simulink model "consigna_5_2"  (R2024b)
settings: Solver=ode45  StartTime=0.0  StopTime=600  FixedStep=1/39789  MaxStep=1e-1  RelTol=1e-5
InitFcn:
  | parametros
values from neighbouring files (symbols this model uses):
  A_corrientes = [0 1; -omega_n_corrientes^2 -2*omega_n_corrientes]    [parametros.m]
  A_inversor = [0 1; -omega_n_inversor^2 -2*omega_n_inversor]    [parametros.m]
  A_posicion = [0 1; -omega_n_posicion^2 -2*omega_n_posicion]    [parametros.m]
  A_temp = -1/20    (= -0.05)    [parametros.m]
  alpha_cu = 3.9 *10^-3    (= 0.0039)    [parametros.m]
  B_corrientes = [0; omega_n_corrientes^2]    [parametros.m]
  B_inversor = [0; omega_n_inversor^2]    [parametros.m]
  b_l = 0.1    [parametros.m]
  b_m = 1.5 * 10^-5    (= 1.5e-05)    [parametros.m]
  B_posicion = [0; omega_n_posicion^2]    [parametros.m]
  B_temp = 1/20    (= 0.05)    [parametros.m]
  ba = J_eq*n*omega_pos    (= 0.0395694444444)    [parametros.m]
  C_corrientes = [1 0]    [parametros.m]
  C_inversor = [1 0]    [parametros.m]
  C_posicion = [1 0]    [parametros.m]
  C_temp = 1    [parametros.m]
  C_ts = 0.818    [parametros.m]
  J_l = (m*l_cm^2 + J_cm) + (m_l * l_l^2)    (= 0.0833)    [parametros.m]
  J_m = 1.4 * 10^-5    (= 1.4e-05)    [parametros.m]
  K_e_int = 3200 ^3    (= 32768000000)    [parametros.m]
  K_e_omega = 3*3200^2    (= 30720000)    [parametros.m]
  K_e_theta = 9600    [parametros.m]
  k_l = m * g * l_cm + m_l * g * l_l    (= 2.4516625)    [parametros.m]
  Ksa = J_eq*n*(omega_pos^2)    (= 31.6555555556)    [parametros.m]
  Ksia = J_eq*(omega_pos^3)    (= 10129.7777778)    [parametros.m]
  L_d = 6.6 * 10^-3    (= 0.0066)    [parametros.m]
  L_ls = 0.8 * 10^-3    (= 0.0008)    [parametros.m]
  L_q = 5.8 * 10^-3    (= 0.0058)    [parametros.m]
  lambda_m = 0.016    [parametros.m]
  P_p = 3    [parametros.m]
  r = 120    [parametros.m]
  R_s_40 = 1.02    [parametros.m]
  R_ts_amb = 146.7    [parametros.m]
  T_sample = 1/f_sample    (= 4.53514739229e-05)    [parametros.m]
  Temp_s_ref = 20    [parametros.m]
  tm = X(1)    [parametros.m]
  tr = X(2)    [parametros.m]
  w1 = 2*pi*r/5    (= 150.796447372)    [parametros.m]
  x0_corrientes = [0;0]    [parametros.m]
  x0_inversor = [0;0]    [parametros.m]
  x0_posicion = [0; 0]    [parametros.m]
  x0_temp = 25    [parametros.m]
libraries: simulink x23, dspsigops x6
(part 2 of 5)

== system consigna_5_2/5.2.5.c ==
  note: CONTROLADOR
  T_per : Inport
  Tº_amb : Inport  Port=2
  q1* : Inport  Port=3
  Calculo rs : Subsystem
  Constant5 : Constant  Value=0
  Controlador PID : Subsystem
  Demux : Demux  Outputs=3
  Desacoplamiento de torque de gravedad : Subsystem
  Desacoplamientos físicos : Subsystem
  Gain5 : Gain  Gain=P_p
  Inversión de tensión : Subsystem
  Modulador de corriente : Subsystem
  Modulador de torque : Subsystem
  Mux : Mux  Inputs=3
  Mux1 : Mux  Inputs=2
  Observador de estado reducido : Subsystem
  Sensores : Subsystem
  Setpoint : Subsystem
  Subsistema físico no lineal : Subsystem
      settings: PortSchema="{\"entries\":[{\"content\":{\"sides\":[{\"content\":{\"connectorIds\":[\"In1\",\"In2\",\"In3\",\"In4\",\"In5\"]},\"type\":\"ConnectorPlacement.EquallySpacedRectSide\",\"uuid\":\"67117692-d9ee-40bf-88b2-d8f6a60dc3b5\"},{\"content\":{\"connectorIds\":[\"Out1\",\"Out2\",\"Out3\"],\"side\":\"RIGHT\"},\"type\":\"ConnectorPlacement.EquallySpacedRectSide\",\"uuid\":\"ca2dbe86-e86f-47c7-8eac-1e82e6a5dbc0\"},{\"content\":{\"connectorIds\":[\"Out4\",\"Out5\",\"Out6\"],\"side\":\"TOP\"},\"type\":\"ConnectorPlacement.EquallySpacedRectSide\",\"uuid\":\"fbd4a5c3-5162-48dd-8002-932f8e6631f6\"}]},\"type\":\"ConnectorPlacement.EquallySpacedConnector\",\"uuid\":\"e55c07f0-88b9-4508-920f-2bf50421126b\"}],\"packageUris\":[\"http://schema.mathworks.com/mf0/Connector/R2020b\"],\"version\":\"1.0\"}"
  TD_PARK : MATLAB Function  TreatAsAtomicUnit=on
  TI_PARK1 : MATLAB Function  TreatAsAtomicUnit=on
  T_l : Outport
  T_m : Outport  Port=2
  "theta_m " : Outport  Port=3
  T_s : Outport  Port=4
  fas : Outport  Port=5
  fbs : Outport  Port=6
  fcs : Outport  Port=7
  v_abcs : Outport  Port=8
  omega_m : Outport  Port=9
  omega_theta_obs : Outport  Port=10
  wires:
  Inversión de tensión/1(v_as) -> Subsistema físico no lineal/2(v_as), Mux/1
  TD_PARK/3(f0s) -> Modulador de corriente/6(i_0s), Desacoplamientos físicos/6(i_0s)  "i_0s"
  TI_PARK1/1(fas) -> Inversión de tensión/1(v_as*)
  Inversión de tensión/2(v_bs) -> Mux/2, Subsistema físico no lineal/3(v_bs)
  TD_PARK/1(fqs) -> Modulador de corriente/4(i_qs), Desacoplamientos físicos/4(i_qs)  "i_qs^r"
  Gain5/1 -> TD_PARK/4(theta_r), TI_PARK1/4(theta_r)
  TI_PARK1/2(fbs) -> Inversión de tensión/2(v_bs*)
  TD_PARK/2(fds) -> Modulador de torque/2(ids), Modulador de corriente/5(i_ds), Desacoplamientos físicos/5(i_ds)  "i_ds^r"
  Desacoplamientos físicos/3(v_0s*') -> TI_PARK1/3(f0s)
  Inversión de tensión/3(v_cs) -> Mux/3, Subsistema físico no lineal/4(v_cs)
  Subsistema físico no lineal/1(theta_m) -> Sensores/1(theta_m)
  Subsistema físico no lineal/2(T_s) -> Sensores/2(T_s)
  Sensores/5(i_cs_medida) -> fcs/1, TD_PARK/3(fcs)
  Demux/1 -> Sensores/3(i_as)
  Modulador de torque/1(iq*) -> Modulador de corriente/1(I_qs*)
  Sensores/4(i_bs_medida) -> fbs/1, TD_PARK/2(fbs)
  Subsistema físico no lineal/5(T_m) -> T_m/1
  Modulador de corriente/1(v_qs*) -> Desacoplamientos físicos/1(v_qs*)
  Constant5/1 -> Modulador de corriente/3(I_0s*), Modulador de corriente/2(I_ds*)
  T_per/1 -> Subsistema físico no lineal/1(T_per)
  Demux/2 -> Sensores/4(i_bs)
  Modulador de corriente/3(v_0s*) -> Desacoplamientos físicos/3(v_0s*)
  Demux/3 -> Sensores/5(i_cs)
  Sensores/1(theta_m_medida) -> "theta_m "/1, Observador de estado reducido/2(theta_m), Gain5/1
  Desacoplamientos físicos/1(v_qs*') -> TI_PARK1/1(fqs)
  Sensores/3(i_as_medida) -> TD_PARK/1(fas), fas/1
  TI_PARK1/3(fcs) -> Inversión de tensión/3(v_cs*)
  Desacoplamientos físicos/2(v_ds*') -> TI_PARK1/2(fds)
  Modulador de corriente/2(v_ds*) -> Desacoplamientos físicos/2(v_ds*)
  Setpoint/2(omega_m*) -> Controlador PID/1(omega_m*)
  q1*/1 -> Setpoint/1(q1*)
  Controlador PID/1(Tm*) -> Observador de estado reducido/1(T_m*), Desacoplamiento de torque de gravedad/1(Tm*)
  Tº_amb/1 -> Subsistema físico no lineal/5(Tº_amb)
  Sensores/2(T_s_medida) -> Calculo rs/1(Ts), T_s/1
  Calculo rs/1(r_s) -> Desacoplamientos físicos/8(r_s)
  Desacoplamiento de torque de gravedad/1(Tm*') -> Modulador de torque/1(Tm*)
  Mux/1 -> v_abcs/1
  Subsistema físico no lineal/4(omega_m) -> omega_m/1  "omega_m"
  Mux1/1 -> omega_theta_obs/1
  Observador de estado reducido/2(theta_m_obs) -> Mux1/2, Desacoplamiento de torque de gravedad/2(theta_m)
  Observador de estado reducido/1(omega_m_obs) -> Mux1/1, Modulador de torque/3(omega_m), Controlador PID/2(omega_m), Desacoplamientos físicos/7(omega_m)
  Subsistema físico no lineal/6(T_l) -> T_l/1
  Subsistema físico no lineal/3(i_abcs) -> Demux/1

== system consigna_5_2/5.2.5.d ==
  note: CONTROLADOR
  T_per : Inport
  Tº_amb : Inport  Port=2
  q1* : Inport  Port=3
  Calculo rs : Subsystem
  Constant5 : Constant  Value=0
  Controlador PID : Subsystem
  Demux : Demux  Outputs=3
  Desacoplamiento de torque de gravedad : Subsystem
  Desacoplamientos físicos : Subsystem
  Gain5 : Gain  Gain=P_p
  Inversión de tensión : Subsystem
  Modulador de corriente : Subsystem
  Modulador de torque : Subsystem
  Mux : Mux  Inputs=3
  Mux1 : Mux  Inputs=2
  Observador de estado reducido : Subsystem
  Sensores : Subsystem
  Setpoint : Subsystem
  Subsistema físico no lineal : Subsystem
      settings: PortSchema="{\"entries\":[{\"content\":{\"sides\":[{\"content\":{\"connectorIds\":[\"In1\",\"In2\",\"In3\",\"In4\",\"In5\"]},\"type\":\"ConnectorPlacement.EquallySpacedRectSide\",\"uuid\":\"67117692-d9ee-40bf-88b2-d8f6a60dc3b5\"},{\"content\":{\"connectorIds\":[\"Out1\",\"Out2\",\"Out3\"],\"side\":\"RIGHT\"},\"type\":\"ConnectorPlacement.EquallySpacedRectSide\",\"uuid\":\"ca2dbe86-e86f-47c7-8eac-1e82e6a5dbc0\"},{\"content\":{\"connectorIds\":[\"Out4\",\"Out5\",\"Out6\"],\"side\":\"TOP\"},\"type\":\"ConnectorPlacement.EquallySpacedRectSide\",\"uuid\":\"fbd4a5c3-5162-48dd-8002-932f8e6631f6\"}]},\"type\":\"ConnectorPlacement.EquallySpacedConnector\",\"uuid\":\"e55c07f0-88b9-4508-920f-2bf50421126b\"}],\"packageUris\":[\"http://schema.mathworks.com/mf0/Connector/R2020b\"],\"version\":\"1.0\"}"
  TD_PARK : MATLAB Function  TreatAsAtomicUnit=on
  TI_PARK1 : MATLAB Function  TreatAsAtomicUnit=on
  T_l : Outport
  T_m : Outport  Port=2
  "theta_m " : Outport  Port=3
  T_s : Outport  Port=4
  fas : Outport  Port=5
  fbs : Outport  Port=6
  fcs : Outport  Port=7
  v_abcs : Outport  Port=8
  omega_theta_obs : Outport  Port=9
  omega_m : Outport  Port=10
  wires:
  Inversión de tensión/1(v_as) -> Subsistema físico no lineal/2(v_as), Mux/1
  TD_PARK/3(f0s) -> Modulador de corriente/6(i_0s), Desacoplamientos físicos/6(i_0s)  "i_0s"
  TI_PARK1/1(fas) -> Inversión de tensión/1(v_as*)
  Inversión de tensión/2(v_bs) -> Subsistema físico no lineal/3(v_bs), Mux/2
  TD_PARK/1(fqs) -> Modulador de corriente/4(i_qs), Desacoplamientos físicos/4(i_qs)  "i_qs^r"
  Gain5/1 -> TD_PARK/4(theta_r), TI_PARK1/4(theta_r)
  TI_PARK1/2(fbs) -> Inversión de tensión/2(v_bs*)
  TD_PARK/2(fds) -> Modulador de torque/2(ids), Modulador de corriente/5(i_ds), Desacoplamientos físicos/5(i_ds)  "i_ds^r"
  Desacoplamientos físicos/3(v_0s*') -> TI_PARK1/3(f0s)
  Inversión de tensión/3(v_cs) -> Subsistema físico no lineal/4(v_cs), Mux/3
  Subsistema físico no lineal/1(theta_m) -> Sensores/1(theta_m)
  Subsistema físico no lineal/2(T_s) -> Sensores/2(T_s)
  Sensores/5(i_cs_medida) -> fcs/1, TD_PARK/3(fcs)
  Demux/1 -> Sensores/3(i_as)
  Modulador de torque/1(iq*) -> Modulador de corriente/1(I_qs*)
  Sensores/4(i_bs_medida) -> fbs/1, TD_PARK/2(fbs)
  Modulador de corriente/1(v_qs*) -> Desacoplamientos físicos/1(v_qs*)
  Constant5/1 -> Modulador de corriente/3(I_0s*), Modulador de corriente/2(I_ds*)
  T_per/1 -> Subsistema físico no lineal/1(T_per)
  Demux/2 -> Sensores/4(i_bs)
  Modulador de corriente/3(v_0s*) -> Desacoplamientos físicos/3(v_0s*)
  Demux/3 -> Sensores/5(i_cs)
  Sensores/1(theta_m_medida) -> "theta_m "/1, Observador de estado reducido/2(theta_m), Gain5/1
  Desacoplamientos físicos/1(v_qs*') -> TI_PARK1/1(fqs)
  Sensores/3(i_as_medida) -> TD_PARK/1(fas), fas/1
  TI_PARK1/3(fcs) -> Inversión de tensión/3(v_cs*)
  Desacoplamientos físicos/2(v_ds*') -> TI_PARK1/2(fds)
  Modulador de corriente/2(v_ds*) -> Desacoplamientos físicos/2(v_ds*)
  Setpoint/2(omega_m*) -> Controlador PID/1(omega_m*)
  q1*/1 -> Setpoint/1(q1*)
  Controlador PID/1(Tm*) -> Observador de estado reducido/1(T_m*), Desacoplamiento de torque de gravedad/1(Tm*)
  Tº_amb/1 -> Subsistema físico no lineal/5(Tº_amb)
  Sensores/2(T_s_medida) -> Calculo rs/1(Ts), T_s/1
  Calculo rs/1(r_s) -> Desacoplamientos físicos/8(r_s)
  Desacoplamiento de torque de gravedad/1(Tm*') -> Modulador de torque/1(Tm*)
  Mux/1 -> v_abcs/1
  Mux1/1 -> omega_theta_obs/1
  Observador de estado reducido/2(theta_m_obs) -> Mux1/2, Desacoplamiento de torque de gravedad/2(theta_m)
  Observador de estado reducido/1(omega_m_obs) -> Mux1/1, Modulador de torque/3(omega_m), Controlador PID/2(omega_m), Desacoplamientos físicos/7(omega_m)
  Subsistema físico no lineal/5(T_m) -> T_m/1
  Subsistema físico no lineal/4(omega_m) -> omega_m/1  "omega_m"
  Subsistema físico no lineal/3(i_abcs) -> Demux/1
  Subsistema físico no lineal/6(T_l) -> T_l/1

== system consigna_5_2/5.2.5.e ==
  note: CONTROLADOR
  T_per : Inport
  Tº_amb : Inport  Port=2
  q1* : Inport  Port=3
  Calculo rs : Subsystem
  Constant5 : Constant  Value=0
  Controlador PID : Subsystem
  Demux : Demux  Outputs=3
  Desacoplamiento de torque de gravedad : Subsystem
  Desacoplamientos físicos : Subsystem
  Gain5 : Gain  Gain=P_p
  Inversión de tensión : Subsystem
  Modulador de corriente : Subsystem
  Modulador de torque : Subsystem
  Mux : Mux  Inputs=3
  Mux1 : Mux  Inputs=2
  Observador de estado reducido : Subsystem
  Sensores : Subsystem
  Setpoint : Subsystem
  Subsistema físico no lineal : Subsystem
      settings: PortSchema="{\"entries\":[{\"content\":{\"sides\":[{\"content\":{\"connectorIds\":[\"In1\",\"In2\",\"In3\",\"In4\",\"In5\"]},\"type\":\"ConnectorPlacement.EquallySpacedRectSide\",\"uuid\":\"67117692-d9ee-40bf-88b2-d8f6a60dc3b5\"},{\"content\":{\"connectorIds\":[\"Out1\",\"Out2\",\"Out3\"],\"side\":\"RIGHT\"},\"type\":\"ConnectorPlacement.EquallySpacedRectSide\",\"uuid\":\"ca2dbe86-e86f-47c7-8eac-1e82e6a5dbc0\"},{\"content\":{\"connectorIds\":[\"Out4\",\"Out5\",\"Out6\"],\"side\":\"TOP\"},\"type\":\"ConnectorPlacement.EquallySpacedRectSide\",\"uuid\":\"fbd4a5c3-5162-48dd-8002-932f8e6631f6\"}]},\"type\":\"ConnectorPlacement.EquallySpacedConnector\",\"uuid\":\"e55c07f0-88b9-4508-920f-2bf50421126b\"}],\"packageUris\":[\"http://schema.mathworks.com/mf0/Connector/R2020b\"],\"version\":\"1.0\"}"
  TD_PARK : MATLAB Function  TreatAsAtomicUnit=on
  TI_PARK1 : MATLAB Function  TreatAsAtomicUnit=on
  T_l : Outport
  T_m : Outport  Port=2
  "theta_m " : Outport  Port=3
  T_s : Outport  Port=4
  fas : Outport  Port=5
  fbs : Outport  Port=6
  fcs : Outport  Port=7
  v_abcs : Outport  Port=8
  omega_theta_obs : Outport  Port=9
  omega_m : Outport  Port=10
  wires:
  Inversión de tensión/1(v_as) -> Subsistema físico no lineal/2(v_as), Mux/1
  TD_PARK/3(f0s) -> Modulador de corriente/6(i_0s), Desacoplamientos físicos/6(i_0s)  "i_0s"
  TI_PARK1/1(fas) -> Inversión de tensión/1(v_as*)
  Inversión de tensión/2(v_bs) -> Subsistema físico no lineal/3(v_bs), Mux/2
  TD_PARK/1(fqs) -> Modulador de corriente/4(i_qs), Desacoplamientos físicos/4(i_qs)  "i_qs^r"
  Gain5/1 -> TD_PARK/4(theta_r), TI_PARK1/4(theta_r)
  TI_PARK1/2(fbs) -> Inversión de tensión/2(v_bs*)
  TD_PARK/2(fds) -> Modulador de torque/2(ids), Modulador de corriente/5(i_ds), Desacoplamientos físicos/5(i_ds)  "i_ds^r"
  Desacoplamientos físicos/3(v_0s*') -> TI_PARK1/3(f0s)
  Inversión de tensión/3(v_cs) -> Subsistema físico no lineal/4(v_cs), Mux/3
  Subsistema físico no lineal/1(theta_m) -> Sensores/1(theta_m)
  Subsistema físico no lineal/2(T_s) -> Sensores/2(T_s)
  Sensores/5(i_cs_medida) -> fcs/1, TD_PARK/3(fcs)
  Modulador de torque/1(iq*) -> Modulador de corriente/1(I_qs*)
  Sensores/4(i_bs_medida) -> fbs/1, TD_PARK/2(fbs)
  Modulador de corriente/1(v_qs*) -> Desacoplamientos físicos/1(v_qs*)
  Constant5/1 -> Modulador de corriente/3(I_0s*), Modulador de corriente/2(I_ds*)
  T_per/1 -> Subsistema físico no lineal/1(T_per)
  Demux/2 -> Sensores/4(i_bs)
  Modulador de corriente/3(v_0s*) -> Desacoplamientos físicos/3(v_0s*)
  Demux/3 -> Sensores/5(i_cs)
  Sensores/1(theta_m_medida) -> "theta_m "/1, Observador de estado reducido/2(theta_m), Gain5/1
  Desacoplamientos físicos/1(v_qs*') -> TI_PARK1/1(fqs)
  Sensores/3(i_as_medida) -> TD_PARK/1(fas), fas/1
  TI_PARK1/3(fcs) -> Inversión de tensión/3(v_cs*)
  Desacoplamientos físicos/2(v_ds*') -> TI_PARK1/2(fds)
  Modulador de corriente/2(v_ds*) -> Desacoplamientos físicos/2(v_ds*)
  Setpoint/2(omega_m*) -> Controlador PID/1(omega_m*)
  q1*/1 -> Setpoint/1(q1*)
  Controlador PID/1(Tm*) -> Observador de estado reducido/1(T_m*), Desacoplamiento de torque de gravedad/1(Tm*)
  Tº_amb/1 -> Subsistema físico no lineal/5(Tº_amb)
  Sensores/2(T_s_medida) -> Calculo rs/1(Ts), T_s/1
  Calculo rs/1(r_s) -> Desacoplamientos físicos/8(r_s)
  Desacoplamiento de torque de gravedad/1(Tm*') -> Modulador de torque/1(Tm*)
  Mux/1 -> v_abcs/1
  Mux1/1 -> omega_theta_obs/1
  Observador de estado reducido/2(theta_m_obs) -> Mux1/2, Desacoplamiento de torque de gravedad/2(theta_m)
  Observador de estado reducido/1(omega_m_obs) -> Mux1/1, Modulador de torque/3(omega_m), Controlador PID/2(omega_m), Desacoplamientos físicos/7(omega_m)
  Subsistema físico no lineal/5(T_m) -> T_m/1
  Subsistema físico no lineal/6(T_l) -> T_l/1
  Subsistema físico no lineal/4(omega_m) -> omega_m/1  "omega_m"
  Subsistema físico no lineal/3(i_abcs) -> Demux/1
  Demux/1 -> Sensores/3(i_as)

== system consigna_5_2/Subsystem ==
  T_per : Inport
  Tº_amb : Inport  Port=2
  q1* : Inport  Port=3
  5.2.6 : Subsystem
  omega_m : Outport
  Tm : Outport  Port=2
  theta_m : Outport  Port=3
  T_s : Outport  Port=4
  i_as : Outport  Port=5
  i_bs : Outport  Port=6
  i_cs : Outport  Port=7
  v_abcs : Outport  Port=8
  omega_theta_obs : Outport  Port=9
  omega_m1 : Outport  Port=10
  wires:
  q1*/1 -> 5.2.6/3(q1*)
  5.2.6/3("theta_m ") -> theta_m/1  "theta_m"
  T_per/1 -> 5.2.6/1(T_per)
  5.2.6/1(T_l) -> omega_m/1  "omega_m"
  5.2.6/4(T_s) -> T_s/1  "T_s"
  5.2.6/2(T_m) -> Tm/1  "Tm"
  5.2.6/5(fas) -> i_as/1  "i_as"
  5.2.6/10(omega_m) -> omega_m1/1  "omega_m"
  5.2.6/9(omega_theta_obs) -> omega_theta_obs/1
  5.2.6/7(fcs) -> i_cs/1  "i_cs"
  Tº_amb/1 -> 5.2.6/2(Tº_amb)
  5.2.6/6(fbs) -> i_bs/1  "i_bs"
  5.2.6/8(v_abcs) -> v_abcs/1

== system consigna_5_2/5.2.1 /Calculo rs ==
  Ts : Inport
  Tamb : Inport  Port=2
  Constant : Constant
  Gain : Gain  Gain=alpha_cu
  Gain1 : Gain  Gain=R_s_40
  Sum : Sum  Inputs=|++
  Sum1 : Sum  Inputs=|-+
  r_s : Outport
  wires:
  Constant/1 -> Sum/1
  Gain/1 -> Sum/2
  Ts/1 -> Sum1/2
  Tamb/1 -> Sum1/1
  Sum1/1 -> Gain/1
  Sum/1 -> Gain1/1
  Gain1/1 -> r_s/1

== system consigna_5_2/5.2.1 /Desacoplamientos físicos ==
  v_qs* : Inport
  v_ds* : Inport  Port=2
  v_0s* : Inport  Port=3
  i_qs : Inport  Port=4
  i_ds : Inport  Port=5
  i_0s : Inport  Port=6
  omega_m : Inport  Port=7
  r_s : Inport  Port=8
  Constant : Constant  Value=lambda_m
  Gain : Gain  Gain=P_p
  Gain1 : Gain  Gain=L_d
  Gain2 : Gain  Gain=L_q*P_p
  Product{,1..4} (5 alike) : Product
  Sum : Sum  Inputs=|++
  Sum1 : Sum  Inputs=|++
  Sum2 : Sum  Inputs=++|
  Sum3 : Sum  Inputs=+-|
  Sum4 : Sum  Inputs=|++
  Sum5 : Sum  Inputs=++|
  v_qs*' : Outport
  v_ds*' : Outport  Port=2
  v_0s*' : Outport  Port=3
  wires:
  Product/1 -> Sum/2
  r_s/1 -> Product4/1, Product/1, Product2/1
  i_qs/1 -> Product/2, Gain2/1
  v_qs*/1 -> Sum/1
  Sum/1 -> Sum1/1
  omega_m/1 -> Product3/2, Gain/1
  Product1/1 -> Sum1/2
  Gain/1 -> Product1/2
  i_ds/1 -> Gain1/1, Product2/2
  Gain1/1 -> Sum2/2
  Constant/1 -> Sum2/1
  Sum2/1 -> Product1/1
  Sum1/1 -> v_qs*'/1
  Product2/1 -> Sum3/1
  Gain2/1 -> Product3/1
  Product3/1 -> Sum3/2
  Sum3/1 -> Sum4/2
  v_ds*/1 -> Sum4/1
  Sum4/1 -> v_ds*'/1
  i_0s/1 -> Product4/2
  Product4/1 -> Sum5/1
  v_0s*/1 -> Sum5/2
  Sum5/1 -> v_0s*'/1

== system consigna_5_2/5.2.1 /Desacoplamientos físicos de torque ==
  Tm* : Inport
  theta_m : Inport  Port=2
  Gain : Gain  Gain=k_l
  Gain1 : Gain  Gain=1/r
  Gain2 : Gain  Gain=1/r
  Sin : Trigonometry
  Sum : Sum  Inputs=|++
  Tm*' : Outport
  wires:
  Tm*/1 -> Sum/1
  theta_m/1 -> Gain1/1
  Sin/1 -> Gain/1
  Sum/1 -> Tm*'/1
  Gain1/1 -> Sin/1
  Gain/1 -> Gain2/1
  Gain2/1 -> Sum/2

== system consigna_5_2/5.2.1 /Modulador de corriente ==
  I_qs* : Inport
  I_ds* : Inport  Port=2
  I_0s* : Inport  Port=3
  i_qs : Inport  Port=4
  i_ds : Inport  Port=5
  i_0s : Inport  Port=6
  Gain : Gain  Gain=5000*L_q
  Gain1 : Gain  Gain=5000*L_d
  Gain2 : Gain  Gain=5000*L_ls
  Sum : Sum  Inputs=+-
  Sum1 : Sum  Inputs=+-
  Sum2 : Sum  Inputs=+-
  v_qs* : Outport
  v_ds* : Outport  Port=2
  v_0s* : Outport  Port=3
  wires:
  Sum2/1 -> Gain2/1
  Sum1/1 -> Gain1/1
  Sum/1 -> Gain/1
  I_qs*/1 -> Sum/1
  i_qs/1 -> Sum/2
  I_ds*/1 -> Sum1/1
  i_ds/1 -> Sum1/2
  I_0s*/1 -> Sum2/1
  i_0s/1 -> Sum2/2
  Gain/1 -> v_qs*/1
  Gain2/1 -> v_0s*/1
  Gain1/1 -> v_ds*/1

== system consigna_5_2/5.2.1 /Modulador de tensión ==
  v_as* : Inport
  v_bs* : Inport  Port=2
  v_cs* : Inport  Port=3
  Gain : Gain
  Gain1 : Gain
  Gain2 : Gain
  v_as : Outport
  v_bs : Outport  Port=2
  v_cs : Outport  Port=3
  wires:
  v_as*/1 -> Gain/1
  Gain/1 -> v_as/1
  v_bs*/1 -> Gain1/1
  Gain1/1 -> v_bs/1
  v_cs*/1 -> Gain2/1
  Gain2/1 -> v_cs/1

== system consigna_5_2/5.2.1 /Modulador de torque ==
  Tm* : Inport
  ids : Inport  Port=2
  omega_m : Inport  Port=3
  Constant : Constant  Value=lambda_m
  Divide : Product  Inputs=/*
  Gain : Gain  Gain=b_m + b_l/r^2
  Gain1 : Gain  Gain=2/(3*P_p)
  Gain2 : Gain  Gain=L_d-L_q
  Sum : Sum  Inputs=|++
  Sum1 : Sum  Inputs=++|
  iq* : Outport
  wires:
  omega_m/1 -> Gain/1
  Sum/1 -> Gain1/1
  ids/1 -> Gain2/1
  Gain2/1 -> Sum1/1
  Constant/1 -> Sum1/2
  Sum1/1 -> Divide/1
  Gain/1 -> Sum/2
  Tm*/1 -> Sum/1
  Gain1/1 -> Divide/2
  Divide/1 -> iq*/1

== system consigna_5_2/5.2.1 /Sensores ==
  theta_m : Inport
  T_s : Inport  Port=2
  i_as : Inport  Port=3
  i_bs : Inport  Port=4
  i_cs : Inport  Port=5
  Gain{,1..4} (5 alike) : Gain
  theta_m_medida : Outport
  T_s_medida : Outport  Port=2
  i_as_medida : Outport  Port=3
  i_bs_medida : Outport  Port=4
  i_cs_medida : Outport  Port=5
  wires:
  theta_m/1 -> Gain/1
  T_s/1 -> Gain1/1
  i_as/1 -> Gain2/1
  Gain/1 -> theta_m_medida/1
  Gain1/1 -> T_s_medida/1
  Gain2/1 -> i_as_medida/1
  Gain3/1 -> i_bs_medida/1
  i_bs/1 -> Gain3/1
  i_cs/1 -> Gain4/1
  Gain4/1 -> i_cs_medida/1

== system consigna_5_2/5.2.1 /Subsistema físico no lineal ==
  note: Retroalimentación natural del torque gravitacional
  T_per : Inport
  v_as : Inport  Port=2
  v_bs : Inport  Port=3
  v_cs : Inport  Port=4
  Tº_amb : Inport  Port=5
  Gain : Gain  Gain=P_p
  Gain1 : Gain  Gain=1/r
  Gain2 : Gain  Gain=k_l
  Mux : Mux  Inputs=3
  Sin : Trigonometry
  Subsistema electromagnético : Subsystem
      settings: PortSchema="{\"entries\":[{\"content\":{\"sides\":[{\"content\":{\"connectorIds\":[\"In1\",\"In2\",\"In3\",\"In4\"]},\"type\":\"ConnectorPlacement.EquallySpacedRectSide\",\"uuid\":\"c9fae60f-a644-4c7d-9a50-e330e891aba8\"},{\"content\":{\"connectorIds\":[\"Out1\",\"Out2\",\"Out3\",\"Out4\"],\"side\":\"RIGHT\"},\"type\":\"ConnectorPlacement.EquallySpacedRectSide\",\"uuid\":\"1bd25713-f5e9-4106-83eb-fb9f8a30d88e\"},{\"content\":{\"connectorIds\":[\"In5\"],\"side\":\"TOP\"},\"type\":\"ConnectorPlacement.EquallySpacedRectSide\",\"uuid\":\"c2f005dd-e04f-426d-b804-ce475aa5422d\"}]},\"type\":\"ConnectorPlacement.EquallySpacedConnector\",\"uuid\":\"9bdc4406-fcef-47cb-a5c0-d4f33f547a91\"}],\"packageUris\":[\"http://schema.mathworks.com/mf0/Connector/R2020b\"],\"version\":\"1.0\"}"
  Subsistema mecánico completo : Subsystem
  Subsistema térmico : Subsystem
  Sum : Sum  Inputs=++|
  TD_PARK : MATLAB Function  TreatAsAtomicUnit=on
  TI_PARK : MATLAB Function  TreatAsAtomicUnit=on
  theta_m : Outport
  T_s : Outport  Port=2
  i_abcs : Outport  Port=3
  omega_m : Outport  Port=4
  T_m : Outport  Port=5
  T_l : Outport  Port=6
  wires:
  Subsistema electromagnético/4(T_m) -> T_m/1, Subsistema mecánico completo/1(T_m)
  Subsistema electromagnético/3(i_0s) -> Subsistema térmico/3(i_0s^r), TI_PARK/3(f0s)
  Subsistema mecánico completo/2(omega_m(t)) -> Subsistema electromagnético/5(omega_m), omega_m/1
  Subsistema electromagnético/1(i_qs^r) -> Subsistema térmico/1(i_qs^r), TI_PARK/1(fqs)
  Subsistema electromagnético/2(i_ds^r) -> Subsistema térmico/2(i_ds^r), TI_PARK/2(fds)
  Sum/1 -> T_l/1, Subsistema mecánico completo/2(T_l)  "T_l"
  TD_PARK/1(fqs) -> Subsistema electromagnético/1(v_qs^r)
  Subsistema mecánico completo/1(theta_m(t)) -> theta_m/1, Gain1/1, Gain/1
  Tº_amb/1 -> Subsistema térmico/4(Tº_amb)
  Mux/1 -> i_abcs/1
  TI_PARK/1(fas) -> Mux/1
  TI_PARK/2(fbs) -> Mux/2
  TI_PARK/3(fcs) -> Mux/3
  v_as/1 -> TD_PARK/1(fas)
  v_cs/1 -> TD_PARK/3(fcs)
  Gain/1 -> TI_PARK/4(theta_r), TD_PARK/4(theta_r)
  v_bs/1 -> TD_PARK/2(fbs)
  Gain1/1 -> Sin/1
  Sin/1 -> Gain2/1
  Gain2/1 -> Sum/1
  T_per/1 -> Sum/2
  TD_PARK/2(fds) -> Subsistema electromagnético/2(v_ds^r)
  TD_PARK/3(f0s) -> Subsistema electromagnético/3(v_0s)
  Subsistema térmico/1(r_s) -> Subsistema electromagnético/4(r_s)
  Subsistema térmico/2(T_s) -> T_s/1

== system consigna_5_2/5.2.3/Calculo rs ==
  Ts : Inport
  Constant : Constant
  Constant1 : Constant  Value=Temp_s_ref
  Gain : Gain  Gain=alpha_cu
  Gain1 : Gain  Gain=R_s_40
  Sum : Sum  Inputs=|++
  Sum1 : Sum  Inputs=|-+
  r_s : Outport
  wires:
  Constant/1 -> Sum/1
  Gain/1 -> Sum/2
  Ts/1 -> Sum1/2
  Constant1/1 -> Sum1/1
  Sum1/1 -> Gain/1
  Sum/1 -> Gain1/1
  Gain1/1 -> r_s/1

== system consigna_5_2/5.2.3/Controlador PID ==
  note: ba: Proporcional al error de velocidad
  note: Ksa: Proporcional a la integral al error de velocidad
  note: Ksia: Porporcional a la doble Integral al error de velocidad
  omega_m* : Inport
  omega_m : Inport  Port=2
  Gain : Gain  Gain=ba
  Gain1 : Gain  Gain=Ksa
  Gain2 : Gain  Gain=Ksia
  Integrator : Integrator
  Integrator1 : Integrator
  Sum : Sum  Inputs=|+-
  Sum1 : Sum  Inputs=+++
  Tm* : Outport
  wires:
  omega_m*/1 -> Sum/1
  omega_m/1 -> Sum/2
  Sum/1 -> Integrator/1, Gain/1
  Integrator/1 -> Integrator1/1, Gain1/1
  Gain/1 -> Sum1/3
  Sum1/1 -> Tm*/1
  Gain1/1 -> Sum1/2
  Integrator1/1 -> Gain2/1
  Gain2/1 -> Sum1/1

== system consigna_5_2/5.2.3/Desacoplamientos físicos ==
  v_qs* : Inport
  v_ds* : Inport  Port=2
  v_0s* : Inport  Port=3
  i_qs : Inport  Port=4
  i_ds : Inport  Port=5
  i_0s : Inport  Port=6
  omega_m : Inport  Port=7
  r_s : Inport  Port=8
  Constant : Constant  Value=lambda_m
  Gain : Gain  Gain=P_p
  Gain1 : Gain  Gain=L_d
  Gain2 : Gain  Gain=L_q*P_p
  Product{,1..4} (5 alike) : Product
  Sum : Sum  Inputs=|++
  Sum1 : Sum  Inputs=|++
  Sum2 : Sum  Inputs=++|
  Sum3 : Sum  Inputs=+-|
  Sum4 : Sum  Inputs=|++
  Sum5 : Sum  Inputs=++|
  v_qs*' : Outport
  v_ds*' : Outport  Port=2
  v_0s*' : Outport  Port=3
  wires:
  Product/1 -> Sum/2
  r_s/1 -> Product4/1, Product/1, Product2/1
  i_qs/1 -> Product/2, Gain2/1
  v_qs*/1 -> Sum/1
  Sum/1 -> Sum1/1
  omega_m/1 -> Product3/2, Gain/1
  Product1/1 -> Sum1/2
  Gain/1 -> Product1/2
  i_ds/1 -> Gain1/1, Product2/2
  Gain1/1 -> Sum2/2
  Constant/1 -> Sum2/1
  Sum2/1 -> Product1/1
  Sum1/1 -> v_qs*'/1
  Product2/1 -> Sum3/1
  Gain2/1 -> Product3/1
  Product3/1 -> Sum3/2
  Sum3/1 -> Sum4/2
  v_ds*/1 -> Sum4/1
  Sum4/1 -> v_ds*'/1
  i_0s/1 -> Product4/2
  Product4/1 -> Sum5/1
  v_0s*/1 -> Sum5/2
  Sum5/1 -> v_0s*'/1

== system consigna_5_2/5.2.3/Desacoplamientos físicos de torque ==
  Tm* : Inport
  theta_m : Inport  Port=2
  Gain : Gain  Gain=k_l
  Gain1 : Gain  Gain=1/r
  Gain2 : Gain  Gain=1/r
  Sin : Trigonometry
  Sum : Sum  Inputs=|++
  Tm*' : Outport
  wires:
  Tm*/1 -> Sum/1
  Sin/1 -> Gain/1
  Sum/1 -> Tm*'/1
  Gain1/1 -> Sin/1
  theta_m/1 -> Gain1/1
  Gain/1 -> Gain2/1
  Gain2/1 -> Sum/2

== system consigna_5_2/5.2.3/Modulador de corriente ==
  I_qs* : Inport
  I_ds* : Inport  Port=2
  I_0s* : Inport  Port=3
  i_qs : Inport  Port=4
  i_ds : Inport  Port=5
  i_0s : Inport  Port=6
  Gain : Gain  Gain=5000*L_q
  Gain1 : Gain  Gain=5000*L_d
  Gain2 : Gain  Gain=5000*L_ls
  Sum : Sum  Inputs=+-
  Sum1 : Sum  Inputs=+-
  Sum2 : Sum  Inputs=+-
  v_qs* : Outport
  v_ds* : Outport  Port=2
  v_0s* : Outport  Port=3
  wires:
  Sum2/1 -> Gain2/1
  Sum1/1 -> Gain1/1
  Sum/1 -> Gain/1
  I_qs*/1 -> Sum/1
  i_qs/1 -> Sum/2
  I_ds*/1 -> Sum1/1
  i_ds/1 -> Sum1/2
  I_0s*/1 -> Sum2/1
  i_0s/1 -> Sum2/2
  Gain/1 -> v_qs*/1
  Gain2/1 -> v_0s*/1
  Gain1/1 -> v_ds*/1

== system consigna_5_2/5.2.3/Modulador de tensión ==
  v_as* : Inport
  v_bs* : Inport  Port=2
  v_cs* : Inport  Port=3
  Gain : Gain
  Gain1 : Gain
  Gain2 : Gain
  v_as : Outport
  v_bs : Outport  Port=2
  v_cs : Outport  Port=3
  wires:
  v_as*/1 -> Gain/1
  Gain/1 -> v_as/1
  v_bs*/1 -> Gain1/1
  Gain1/1 -> v_bs/1
  v_cs*/1 -> Gain2/1
  Gain2/1 -> v_cs/1

== system consigna_5_2/5.2.3/Modulador de torque ==
  Tm* : Inport
  ids : Inport  Port=2
  omega_m : Inport  Port=3
  Constant : Constant  Value=lambda_m
  Divide : Product  Inputs=/*
  Gain : Gain  Gain=b_m + b_l/r^2
  Gain1 : Gain  Gain=2/(3*P_p)
  Gain2 : Gain  Gain=L_d-L_q
  Sum : Sum  Inputs=|++
  Sum1 : Sum  Inputs=++|
  iq* : Outport
  wires:
  omega_m/1 -> Gain/1
  Sum/1 -> Gain1/1
  ids/1 -> Gain2/1
  Gain2/1 -> Sum1/1
  Constant/1 -> Sum1/2
  Sum1/1 -> Divide/1
  Gain/1 -> Sum/2
  Tm*/1 -> Sum/1
  Gain1/1 -> Divide/2
  Divide/1 -> iq*/1

== system consigna_5_2/5.2.3/Observador de estado reducido ==
  T_m* : Inport
  theta_m : Inport  Port=2
  Gain : Gain  Gain=1/(J_m+(J_l/r^2))
  Gain1 : Gain  Gain=K_e_theta
  Gain2 : Gain  Gain=K_e_omega
  Integrator : Integrator
  Integrator1 : Integrator
  Sum : Sum  Inputs=|++
  Sum1 : Sum  Inputs=|++
  Sum2 : Sum  Inputs=|-+
  omega_m_obs : Outport
  theta_m_obs : Outport  Port=2
  wires:
  T_m*/1 -> Gain/1
  Gain/1 -> Sum/1
  Sum/1 -> Integrator/1
  Integrator1/1 -> theta_m_obs/1, Sum2/1
  Integrator/1 -> Sum1/1
  Sum1/1 -> omega_m_obs/1, Integrator1/1
  theta_m/1 -> Sum2/2
  Gain1/1 -> Sum1/2
  Sum2/1 -> Gain2/1, Gain1/1
  Gain2/1 -> Sum/2

== system consigna_5_2/5.2.3/Sensores ==
  theta_m : Inport
  T_s : Inport  Port=2
  i_as : Inport  Port=3
  i_bs : Inport  Port=4
  i_cs : Inport  Port=5
  Gain{,1..4} (5 alike) : Gain
  theta_m_medida : Outport
  T_s_medida : Outport  Port=2
  i_as_medida : Outport  Port=3
  i_bs_medida : Outport  Port=4
  i_cs_medida : Outport  Port=5
  wires:
  theta_m/1 -> Gain/1
  T_s/1 -> Gain1/1
  i_as/1 -> Gain2/1
  Gain/1 -> theta_m_medida/1
  Gain1/1 -> T_s_medida/1
  Gain2/1 -> i_as_medida/1
  Gain3/1 -> i_bs_medida/1
  i_bs/1 -> Gain3/1
  i_cs/1 -> Gain4/1
  Gain4/1 -> i_cs_medida/1

== system consigna_5_2/5.2.3/Setpoint ==
  q1* : Inport
  Derivative : Derivative
  Gain : Gain  Gain=r
  theta_m* : Outport
  omega_m* : Outport  Port=2
  wires:
  q1*/1 -> Gain/1
  Gain/1 -> Derivative/1, theta_m*/1
  Derivative/1 -> omega_m*/1

== system consigna_5_2/5.2.3/Subsistema físico no lineal ==
  note: Retroalimentación natural del torque gravitacional
  T_per : Inport
  v_as : Inport  Port=2
  v_bs : Inport  Port=3
  v_cs : Inport  Port=4
  Tº_amb : Inport  Port=5
  Gain : Gain  Gain=P_p
  Gain1 : Gain  Gain=1/r
  Gain2 : Gain  Gain=k_l
  Mux : Mux  Inputs=3
  Scope : Scope
  Sin : Trigonometry
  Subsistema electromagnético : Subsystem
      settings: PortSchema="{\"entries\":[{\"content\":{\"sides\":[{\"content\":{\"connectorIds\":[\"In1\",\"In2\",\"In3\",\"In4\"]},\"type\":\"ConnectorPlacement.EquallySpacedRectSide\",\"uuid\":\"c9fae60f-a644-4c7d-9a50-e330e891aba8\"},{\"content\":{\"connectorIds\":[\"Out1\",\"Out2\",\"Out3\",\"Out4\"],\"side\":\"RIGHT\"},\"type\":\"ConnectorPlacement.EquallySpacedRectSide\",\"uuid\":\"1bd25713-f5e9-4106-83eb-fb9f8a30d88e\"},{\"content\":{\"connectorIds\":[\"In5\"],\"side\":\"TOP\"},\"type\":\"ConnectorPlacement.EquallySpacedRectSide\",\"uuid\":\"c2f005dd-e04f-426d-b804-ce475aa5422d\"}]},\"type\":\"ConnectorPlacement.EquallySpacedConnector\",\"uuid\":\"9bdc4406-fcef-47cb-a5c0-d4f33f547a91\"}],\"packageUris\":[\"http://schema.mathworks.com/mf0/Connector/R2020b\"],\"version\":\"1.0\"}"
  Subsistema mecánico completo : Subsystem
  Subsistema térmico : Subsystem
  Sum : Sum  Inputs=++|
  TD_PARK : MATLAB Function  TreatAsAtomicUnit=on
  TI_PARK : MATLAB Function  TreatAsAtomicUnit=on
  theta_m : Outport
  T_s : Outport  Port=2
  i_abcs : Outport  Port=3
  omega_m : Outport  Port=4
  T_m : Outport  Port=5
  T_l : Outport  Port=6
  wires:
  Subsistema electromagnético/4(T_m) -> T_m/1, Subsistema mecánico completo/1(T_m)
  Subsistema electromagnético/3(i_0s) -> Subsistema térmico/3(i_0s^r), TI_PARK/3(f0s)
  Subsistema mecánico completo/2(omega_m(t)) -> Subsistema electromagnético/5(omega_m), Scope/1, omega_m/1
  Subsistema electromagnético/1(i_qs^r) -> Subsistema térmico/1(i_qs^r), TI_PARK/1(fqs)
  Subsistema electromagnético/2(i_ds^r) -> Subsistema térmico/2(i_ds^r), TI_PARK/2(fds)
  Sum/1 -> T_l/1, Subsistema mecánico completo/2(T_l)  "T_l"
  TD_PARK/1(fqs) -> Subsistema electromagnético/1(v_qs^r)
  Tº_amb/1 -> Subsistema térmico/4(Tº_amb)
  Mux/1 -> i_abcs/1
  TI_PARK/1(fas) -> Mux/1
  TI_PARK/2(fbs) -> Mux/2
  TI_PARK/3(fcs) -> Mux/3
  v_as/1 -> TD_PARK/1(fas)
  v_cs/1 -> TD_PARK/3(fcs)
  Gain/1 -> TI_PARK/4(theta_r), TD_PARK/4(theta_r)
  v_bs/1 -> TD_PARK/2(fbs)
  Gain1/1 -> Sin/1
  Sin/1 -> Gain2/1
  Gain2/1 -> Sum/1
  T_per/1 -> Sum/2
  TD_PARK/2(fds) -> Subsistema electromagnético/2(v_ds^r)
  TD_PARK/3(f0s) -> Subsistema electromagnético/3(v_0s)
  Subsistema térmico/1(r_s) -> Subsistema electromagnético/4(r_s)
  Subsistema térmico/2(T_s) -> T_s/1
  Subsistema mecánico completo/1(theta_m(t)) -> theta_m/1, Gain1/1, Gain/1

== system consigna_5_2/5.2.4/Calculo rs ==
  Ts : Inport
  Constant : Constant
  Constant1 : Constant  Value=Temp_s_ref
  Gain : Gain  Gain=alpha_cu
  Gain1 : Gain  Gain=R_s_40
  Sum : Sum  Inputs=|++
  Sum1 : Sum  Inputs=|-+
  r_s : Outport
  wires:
  Constant/1 -> Sum/1
  Gain/1 -> Sum/2
  Ts/1 -> Sum1/2
  Constant1/1 -> Sum1/1
  Sum1/1 -> Gain/1
  Sum/1 -> Gain1/1
  Gain1/1 -> r_s/1

== system consigna_5_2/5.2.4/Controlador PID ==
  note: ba: Proporcional al error de velocidad
  note: Ksa: Proporcional a la integral al error de velocidad
  note: Ksia: Porporcional a la doble Integral al error de velocidad
  omega_m* : Inport
  omega_m : Inport  Port=2
  Gain : Gain  Gain=ba
  Gain1 : Gain  Gain=Ksa
  Gain2 : Gain  Gain=Ksia
  Integrator : Integrator
  Integrator1 : Integrator
  Sum : Sum  Inputs=|+-
  Sum1 : Sum  Inputs=+++
  Tm* : Outport
  wires:
  omega_m*/1 -> Sum/1
  omega_m/1 -> Sum/2
  Sum/1 -> Integrator/1, Gain/1
  Integrator/1 -> Integrator1/1, Gain1/1
  Gain/1 -> Sum1/3
  Sum1/1 -> Tm*/1
  Gain1/1 -> Sum1/2
  Integrator1/1 -> Gain2/1
  Gain2/1 -> Sum1/1

== system consigna_5_2/5.2.4/Desacoplamiento de torque de gravedad ==
  Tm* : Inport
  theta_m : Inport  Port=2
  Gain : Gain  Gain=k_l
  Gain1 : Gain  Gain=1/r
  Gain2 : Gain  Gain=1/r
  Sin : Trigonometry
  Sum : Sum  Inputs=|++
  Tm*' : Outport
  wires:
  Tm*/1 -> Sum/1
  Sin/1 -> Gain/1
  Sum/1 -> Tm*'/1
  Gain1/1 -> Sin/1
  theta_m/1 -> Gain1/1
  Gain/1 -> Gain2/1
  Gain2/1 -> Sum/2

== system consigna_5_2/5.2.4/Desacoplamientos físicos ==
  v_qs* : Inport
  v_ds* : Inport  Port=2
  v_0s* : Inport  Port=3
  i_qs : Inport  Port=4
  i_ds : Inport  Port=5
  i_0s : Inport  Port=6
  omega_m : Inport  Port=7
  r_s : Inport  Port=8
  Constant : Constant  Value=lambda_m
  Gain : Gain  Gain=P_p
  Gain1 : Gain  Gain=L_d
  Gain2 : Gain  Gain=L_q*P_p
  Product{,1..4} (5 alike) : Product
  Sum : Sum  Inputs=|++
  Sum1 : Sum  Inputs=|++
  Sum2 : Sum  Inputs=++|
  Sum3 : Sum  Inputs=+-|
  Sum4 : Sum  Inputs=|++
  Sum5 : Sum  Inputs=++|
  v_qs*' : Outport
  v_ds*' : Outport  Port=2
  v_0s*' : Outport  Port=3
  wires:
  Product/1 -> Sum/2
  r_s/1 -> Product4/1, Product/1, Product2/1
  i_qs/1 -> Product/2, Gain2/1
  v_qs*/1 -> Sum/1
  Sum/1 -> Sum1/1
  omega_m/1 -> Product3/2, Gain/1
  Product1/1 -> Sum1/2
  Gain/1 -> Product1/2
  i_ds/1 -> Gain1/1, Product2/2
  Gain1/1 -> Sum2/2
  Constant/1 -> Sum2/1
  Sum2/1 -> Product1/1
  Sum1/1 -> v_qs*'/1
  Product2/1 -> Sum3/1
  Gain2/1 -> Product3/1
  Product3/1 -> Sum3/2
  Sum3/1 -> Sum4/2
  v_ds*/1 -> Sum4/1
  Sum4/1 -> v_ds*'/1
  i_0s/1 -> Product4/2
  Product4/1 -> Sum5/1
  v_0s*/1 -> Sum5/2
  Sum5/1 -> v_0s*'/1

== system consigna_5_2/5.2.4/Inversión de tensión ==
  v_as* : Inport
  v_bs* : Inport  Port=2
  v_cs* : Inport  Port=3
  Gain : Gain
  Gain1 : Gain
  Gain2 : Gain
  Saturation : Saturate  Commented=on  UpperLimit=20  LowerLimit=-20
  Saturation1 : Saturate  Commented=on  UpperLimit=20  LowerLimit=-20
  Saturation2 : Saturate  Commented=on  UpperLimit=20  LowerLimit=-20
  v_as : Outport
  v_bs : Outport  Port=2
  v_cs : Outport  Port=3
  wires:
  v_as*/1 -> Gain/1
  v_bs*/1 -> Gain1/1
  v_cs*/1 -> Gain2/1
  Gain/1 -> v_as/1
  Gain1/1 -> v_bs/1
  Gain2/1 -> v_cs/1

== system consigna_5_2/5.2.4/Modulador de corriente ==
  I_qs* : Inport
  I_ds* : Inport  Port=2
  I_0s* : Inport  Port=3
  i_qs : Inport  Port=4
  i_ds : Inport  Port=5
  i_0s : Inport  Port=6
  Gain : Gain  Gain=5000*L_q
  Gain1 : Gain  Gain=5000*L_d
  Gain2 : Gain  Gain=5000*L_ls
  Sum : Sum  Inputs=+-
  Sum1 : Sum  Inputs=+-
  Sum2 : Sum  Inputs=+-
  v_qs* : Outport
  v_ds* : Outport  Port=2
  v_0s* : Outport  Port=3
  wires:
  Sum2/1 -> Gain2/1
  Sum1/1 -> Gain1/1
  Sum/1 -> Gain/1
  I_qs*/1 -> Sum/1
  i_qs/1 -> Sum/2
  I_ds*/1 -> Sum1/1
  i_ds/1 -> Sum1/2
  I_0s*/1 -> Sum2/1
  i_0s/1 -> Sum2/2
  Gain/1 -> v_qs*/1
  Gain2/1 -> v_0s*/1
  Gain1/1 -> v_ds*/1

== system consigna_5_2/5.2.4/Modulador de torque ==
  Tm* : Inport
  ids : Inport  Port=2
  omega_m : Inport  Port=3
  Constant : Constant  Value=lambda_m
  Divide : Product  Inputs=/*
  Gain : Gain  Gain=b_m + b_l/r^2
  Gain1 : Gain  Gain=2/(3*P_p)
  Gain2 : Gain  Gain=L_d-L_q
  Sum : Sum  Inputs=|++
  Sum1 : Sum  Inputs=++|
  iq* : Outport
  wires:
  omega_m/1 -> Gain/1
  Sum/1 -> Gain1/1
  ids/1 -> Gain2/1
  Gain2/1 -> Sum1/1
  Constant/1 -> Sum1/2
  Sum1/1 -> Divide/1
  Gain/1 -> Sum/2
  Tm*/1 -> Sum/1
  Gain1/1 -> Divide/2
  Divide/1 -> iq*/1

== system consigna_5_2/5.2.4/Observador de estado reducido ==
  T_m* : Inport
  theta_m : Inport  Port=2
  Gain : Gain  Gain=1/(J_m+(J_l/r^2))
  Gain1 : Gain  Gain=6400
  Gain2 : Gain  Gain=10240000
  Integrator : Integrator
  Integrator1 : Integrator
  Sum : Sum  Inputs=|++
  Sum1 : Sum  Inputs=|++
  Sum2 : Sum  Inputs=|-+
  omega_m_obs : Outport
  theta_m_obs : Outport  Port=2
  wires:
  T_m*/1 -> Gain/1
  Gain/1 -> Sum/1
  Sum/1 -> Integrator/1
  Integrator1/1 -> theta_m_obs/1, Sum2/1
  Integrator/1 -> Sum1/1
  Sum1/1 -> omega_m_obs/1, Integrator1/1
  theta_m/1 -> Sum2/2
  Gain1/1 -> Sum1/2
  Sum2/1 -> Gain2/1, Gain1/1
  Gain2/1 -> Sum/2

== system consigna_5_2/5.2.4/Sensores ==
  theta_m : Inport
  T_s : Inport  Port=2
  i_as : Inport  Port=3
  i_bs : Inport  Port=4
  i_cs : Inport  Port=5
  Gain{,1..4} (5 alike) : Gain
  theta_m_medida : Outport
  T_s_medida : Outport  Port=2
  i_as_medida : Outport  Port=3
  i_bs_medida : Outport  Port=4
  i_cs_medida : Outport  Port=5
  wires:
  theta_m/1 -> Gain/1
  T_s/1 -> Gain1/1
  i_as/1 -> Gain2/1
  Gain/1 -> theta_m_medida/1
  Gain1/1 -> T_s_medida/1
  Gain2/1 -> i_as_medida/1
  Gain3/1 -> i_bs_medida/1
  i_bs/1 -> Gain3/1
  i_cs/1 -> Gain4/1
  Gain4/1 -> i_cs_medida/1

== system consigna_5_2/5.2.4/Setpoint ==
  q1* : Inport
  Derivative : Derivative
  Gain : Gain  Gain=r
  theta_m* : Outport
  omega_m* : Outport  Port=2
  wires:
  q1*/1 -> Gain/1
  Gain/1 -> Derivative/1, theta_m*/1
  Derivative/1 -> omega_m*/1

== system consigna_5_2/5.2.4/Subsistema físico no lineal ==
  note: Retroalimentación natural del torque gravitacional
  T_per : Inport
  v_as : Inport  Port=2
  v_bs : Inport  Port=3
  v_cs : Inport  Port=4
  Tº_amb : Inport  Port=5
  Gain : Gain  Gain=P_p
  Gain1 : Gain  Gain=1/r
  Gain2 : Gain  Gain=k_l
  Mux : Mux  Inputs=3
  Scope : Scope
  Sin : Trigonometry
  Subsistema electromagnético : Subsystem
      settings: PortSchema="{\"entries\":[{\"content\":{\"sides\":[{\"content\":{\"connectorIds\":[\"In1\",\"In2\",\"In3\",\"In4\"]},\"type\":\"ConnectorPlacement.EquallySpacedRectSide\",\"uuid\":\"c9fae60f-a644-4c7d-9a50-e330e891aba8\"},{\"content\":{\"connectorIds\":[\"Out1\",\"Out2\",\"Out3\",\"Out4\"],\"side\":\"RIGHT\"},\"type\":\"ConnectorPlacement.EquallySpacedRectSide\",\"uuid\":\"1bd25713-f5e9-4106-83eb-fb9f8a30d88e\"},{\"content\":{\"connectorIds\":[\"In5\"],\"side\":\"TOP\"},\"type\":\"ConnectorPlacement.EquallySpacedRectSide\",\"uuid\":\"c2f005dd-e04f-426d-b804-ce475aa5422d\"}]},\"type\":\"ConnectorPlacement.EquallySpacedConnector\",\"uuid\":\"9bdc4406-fcef-47cb-a5c0-d4f33f547a91\"}],\"packageUris\":[\"http://schema.mathworks.com/mf0/Connector/R2020b\"],\"version\":\"1.0\"}"
  Subsistema mecánico completo : Subsystem
  Subsistema térmico : Subsystem
  Sum : Sum  Inputs=++|
  TD_PARK : MATLAB Function  TreatAsAtomicUnit=on
  TI_PARK : MATLAB Function  TreatAsAtomicUnit=on
  theta_m : Outport
  T_s : Outport  Port=2
  i_abcs : Outport  Port=3
  omega_m : Outport  Port=4
  T_m : Outport  Port=5
  T_l : Outport  Port=6
  wires:
  Subsistema electromagnético/4(T_m) -> T_m/1, Subsistema mecánico completo/1(T_m)
  Subsistema electromagnético/3(i_0s) -> Subsistema térmico/3(i_0s^r), TI_PARK/3(f0s)
  Subsistema mecánico completo/2(omega_m(t)) -> Subsistema electromagnético/5(omega_m), Scope/1, omega_m/1
  Subsistema electromagnético/1(i_qs^r) -> Subsistema térmico/1(i_qs^r), TI_PARK/1(fqs)
  Subsistema electromagnético/2(i_ds^r) -> Subsistema térmico/2(i_ds^r), TI_PARK/2(fds)
  Sum/1 -> T_l/1, Subsistema mecánico completo/2(T_l)  "T_l"
  TD_PARK/1(fqs) -> Subsistema electromagnético/1(v_qs^r)
  Tº_amb/1 -> Subsistema térmico/4(Tº_amb)
  Mux/1 -> i_abcs/1
  TI_PARK/1(fas) -> Mux/1
  TI_PARK/2(fbs) -> Mux/2
  TI_PARK/3(fcs) -> Mux/3
  v_as/1 -> TD_PARK/1(fas)
  v_cs/1 -> TD_PARK/3(fcs)
  Gain/1 -> TI_PARK/4(theta_r), TD_PARK/4(theta_r)
  v_bs/1 -> TD_PARK/2(fbs)
  Gain1/1 -> Sin/1
  Sin/1 -> Gain2/1
  Gain2/1 -> Sum/1
  T_per/1 -> Sum/2
  TD_PARK/2(fds) -> Subsistema electromagnético/2(v_ds^r)
  TD_PARK/3(f0s) -> Subsistema electromagnético/3(v_0s)
  Subsistema térmico/1(r_s) -> Subsistema electromagnético/4(r_s)
  Subsistema térmico/2(T_s) -> T_s/1
  Subsistema mecánico completo/1(theta_m(t)) -> theta_m/1, Gain1/1, Gain/1

== system consigna_5_2/5.2.4.b/Calculo rs ==
  Ts : Inport
  Constant : Constant
  Constant1 : Constant  Value=Temp_s_ref
  Gain : Gain  Gain=alpha_cu
  Gain1 : Gain  Gain=R_s_40
  Sum : Sum  Inputs=|++
  Sum1 : Sum  Inputs=|-+
  r_s : Outport
  wires:
  Constant/1 -> Sum/1
  Gain/1 -> Sum/2
  Ts/1 -> Sum1/2
  Constant1/1 -> Sum1/1
  Sum1/1 -> Gain/1
  Sum/1 -> Gain1/1
  Gain1/1 -> r_s/1

== system consigna_5_2/5.2.4.b/Controlador PID ==
  note: ba: Proporcional al error de velocidad
  note: Ksa: Proporcional a la integral al error de velocidad
  note: Ksia: Porporcional a la doble Integral al error de velocidad
  omega_m* : Inport
  omega_m : Inport  Port=2
  Gain : Gain  Gain=ba
  Gain1 : Gain  Gain=Ksa
  Gain2 : Gain  Gain=Ksia
  Integrator : Integrator
  Integrator1 : Integrator
  Sum : Sum  Inputs=|+-
  Sum1 : Sum  Inputs=+++
  Tm* : Outport
  wires:
  omega_m*/1 -> Sum/1
  omega_m/1 -> Sum/2
  Sum/1 -> Integrator/1, Gain/1
  Integrator/1 -> Integrator1/1, Gain1/1
  Gain/1 -> Sum1/3
  Sum1/1 -> Tm*/1
  Gain1/1 -> Sum1/2
  Integrator1/1 -> Gain2/1
  Gain2/1 -> Sum1/1

== system consigna_5_2/5.2.4.b/Desacoplamiento de torque de gravedad ==
  Tm* : Inport
  theta_m : Inport  Port=2
  Gain : Gain  Gain=k_l
  Gain1 : Gain  Gain=1/r
  Gain2 : Gain  Gain=1/r
  Sin : Trigonometry
  Sum : Sum  Inputs=|++
  Tm*' : Outport
  wires:
  Tm*/1 -> Sum/1
  Sin/1 -> Gain/1
  Sum/1 -> Tm*'/1
  Gain1/1 -> Sin/1
  theta_m/1 -> Gain1/1
  Gain/1 -> Gain2/1
  Gain2/1 -> Sum/2

== system consigna_5_2/5.2.4.b/Desacoplamientos físicos ==
  v_qs* : Inport
  v_ds* : Inport  Port=2
  v_0s* : Inport  Port=3
  i_qs : Inport  Port=4
  i_ds : Inport  Port=5
  i_0s : Inport  Port=6
  omega_m : Inport  Port=7
  r_s : Inport  Port=8
  Constant : Constant  Value=lambda_m
  Gain : Gain  Gain=P_p
  Gain1 : Gain  Gain=L_d
  Gain2 : Gain  Gain=L_q*P_p
  Product{,1..4} (5 alike) : Product
  Sum : Sum  Inputs=|++
  Sum1 : Sum  Inputs=|++
  Sum2 : Sum  Inputs=++|
  Sum3 : Sum  Inputs=+-|
  Sum4 : Sum  Inputs=|++
  Sum5 : Sum  Inputs=++|
  v_qs*' : Outport
  v_ds*' : Outport  Port=2
  v_0s*' : Outport  Port=3
  wires:
  Product/1 -> Sum/2
  r_s/1 -> Product4/1, Product/1, Product2/1
  i_qs/1 -> Product/2, Gain2/1
  v_qs*/1 -> Sum/1
  Sum/1 -> Sum1/1
  omega_m/1 -> Product3/2, Gain/1
  Product1/1 -> Sum1/2
  Gain/1 -> Product1/2
  i_ds/1 -> Gain1/1, Product2/2
  Gain1/1 -> Sum2/2
  Constant/1 -> Sum2/1
  Sum2/1 -> Product1/1
  Sum1/1 -> v_qs*'/1
  Product2/1 -> Sum3/1
  Gain2/1 -> Product3/1
  Product3/1 -> Sum3/2
  Sum3/1 -> Sum4/2
  v_ds*/1 -> Sum4/1
  Sum4/1 -> v_ds*'/1
  i_0s/1 -> Product4/2
  Product4/1 -> Sum5/1
  v_0s*/1 -> Sum5/2
  Sum5/1 -> v_0s*'/1

== system consigna_5_2/5.2.4.b/Inversión de tensión ==
  v_as* : Inport
  v_bs* : Inport  Port=2
  v_cs* : Inport  Port=3
  Gain : Gain
  Gain1 : Gain
  Gain2 : Gain
  Saturation : Saturate  Commented=on  UpperLimit=20  LowerLimit=-20
  Saturation1 : Saturate  Commented=on  UpperLimit=20  LowerLimit=-20
  Saturation2 : Saturate  Commented=on  UpperLimit=20  LowerLimit=-20
  v_as : Outport
  v_bs : Outport  Port=2
  v_cs : Outport  Port=3
  wires:
  v_as*/1 -> Gain/1
  v_bs*/1 -> Gain1/1
  v_cs*/1 -> Gain2/1
  Gain/1 -> v_as/1
  Gain1/1 -> v_bs/1
  Gain2/1 -> v_cs/1

== system consigna_5_2/5.2.4.b/Modulador de corriente ==
  I_qs* : Inport
  I_ds* : Inport  Port=2
  I_0s* : Inport  Port=3
  i_qs : Inport  Port=4
  i_ds : Inport  Port=5
  i_0s : Inport  Port=6
  Gain : Gain  Gain=5000*L_q
  Gain1 : Gain  Gain=5000*L_d
  Gain2 : Gain  Gain=5000*L_ls
  Sum : Sum  Inputs=+-
  Sum1 : Sum  Inputs=+-
  Sum2 : Sum  Inputs=+-
  v_qs* : Outport
  v_ds* : Outport  Port=2
  v_0s* : Outport  Port=3
  wires:
  Sum2/1 -> Gain2/1
  Sum1/1 -> Gain1/1
  Sum/1 -> Gain/1
  I_qs*/1 -> Sum/1
  i_qs/1 -> Sum/2
  I_ds*/1 -> Sum1/1
  i_ds/1 -> Sum1/2
  I_0s*/1 -> Sum2/1
  i_0s/1 -> Sum2/2
  Gain/1 -> v_qs*/1
  Gain2/1 -> v_0s*/1
  Gain1/1 -> v_ds*/1

== system consigna_5_2/5.2.4.b/Modulador de torque ==
  Tm* : Inport
  ids : Inport  Port=2
  omega_m : Inport  Port=3
  Constant : Constant  Value=lambda_m
  Divide : Product  Inputs=/*
  Gain : Gain  Gain=b_m + b_l/r^2
  Gain1 : Gain  Gain=2/(3*P_p)
  Gain2 : Gain  Gain=L_d-L_q
  Sum : Sum  Inputs=|++
  Sum1 : Sum  Inputs=++|
  iq* : Outport
  wires:
  omega_m/1 -> Gain/1
  Sum/1 -> Gain1/1
  ids/1 -> Gain2/1
  Gain2/1 -> Sum1/1
  Constant/1 -> Sum1/2
  Sum1/1 -> Divide/1
  Gain/1 -> Sum/2
  Tm*/1 -> Sum/1
  Gain1/1 -> Divide/2
  Divide/1 -> iq*/1

== system consigna_5_2/5.2.4.b/Observador de estado reducido ==
  T_m* : Inport
  theta_m : Inport  Port=2
  Gain : Gain  Gain=1/(J_m+(J_l/r^2))
  Gain1 : Gain  Gain=K_e_theta
  Gain2 : Gain  Gain=K_e_omega
  Integrator : Integrator
  Integrator1 : Integrator
  Sum : Sum  Inputs=|++
  Sum1 : Sum  Inputs=|++
  Sum2 : Sum  Inputs=|-+
  omega_m_obs : Outport
  theta_m_obs : Outport  Port=2
  wires:
  T_m*/1 -> Gain/1
  Gain/1 -> Sum/1
  Sum/1 -> Integrator/1
  Integrator1/1 -> theta_m_obs/1, Sum2/1
  Integrator/1 -> Sum1/1
  Sum1/1 -> omega_m_obs/1, Integrator1/1
  theta_m/1 -> Sum2/2
  Gain1/1 -> Sum1/2
  Sum2/1 -> Gain2/1, Gain1/1
  Gain2/1 -> Sum/2

== system consigna_5_2/5.2.4.b/Sensores ==
  theta_m : Inport
  T_s : Inport  Port=2
  i_as : Inport  Port=3
  i_bs : Inport  Port=4
  i_cs : Inport  Port=5
  Gain{,1..4} (5 alike) : Gain
  theta_m_medida : Outport
  T_s_medida : Outport  Port=2
  i_as_medida : Outport  Port=3
  i_bs_medida : Outport  Port=4
  i_cs_medida : Outport  Port=5
  wires:
  theta_m/1 -> Gain/1
  T_s/1 -> Gain1/1
  i_as/1 -> Gain2/1
  Gain/1 -> theta_m_medida/1
  Gain1/1 -> T_s_medida/1
  Gain2/1 -> i_as_medida/1
  Gain3/1 -> i_bs_medida/1
  i_bs/1 -> Gain3/1
  i_cs/1 -> Gain4/1
  Gain4/1 -> i_cs_medida/1

== system consigna_5_2/5.2.4.b/Setpoint ==
  q1* : Inport
  Derivative : Derivative
  Gain : Gain  Gain=r
  theta_m* : Outport
  omega_m* : Outport  Port=2
  wires:
  q1*/1 -> Gain/1
  Gain/1 -> theta_m*/1, Derivative/1
  Derivative/1 -> omega_m*/1

== system consigna_5_2/5.2.4.b/Subsistema físico no lineal ==
  note: Retroalimentación natural del torque gravitacional
  T_per : Inport
  v_as : Inport  Port=2
  v_bs : Inport  Port=3
  v_cs : Inport  Port=4
  Tº_amb : Inport  Port=5
  Gain : Gain  Gain=P_p
  Gain1 : Gain  Gain=1/r
  Gain2 : Gain  Gain=k_l
  Mux : Mux  Inputs=3
  Scope : Scope
  Sin : Trigonometry
  Subsistema electromagnético : Subsystem
      settings: PortSchema="{\"entries\":[{\"content\":{\"sides\":[{\"content\":{\"connectorIds\":[\"In1\",\"In2\",\"In3\",\"In4\"]},\"type\":\"ConnectorPlacement.EquallySpacedRectSide\",\"uuid\":\"c9fae60f-a644-4c7d-9a50-e330e891aba8\"},{\"content\":{\"connectorIds\":[\"Out1\",\"Out2\",\"Out3\",\"Out4\"],\"side\":\"RIGHT\"},\"type\":\"ConnectorPlacement.EquallySpacedRectSide\",\"uuid\":\"1bd25713-f5e9-4106-83eb-fb9f8a30d88e\"},{\"content\":{\"connectorIds\":[\"In5\"],\"side\":\"TOP\"},\"type\":\"ConnectorPlacement.EquallySpacedRectSide\",\"uuid\":\"c2f005dd-e04f-426d-b804-ce475aa5422d\"}]},\"type\":\"ConnectorPlacement.EquallySpacedConnector\",\"uuid\":\"9bdc4406-fcef-47cb-a5c0-d4f33f547a91\"}],\"packageUris\":[\"http://schema.mathworks.com/mf0/Connector/R2020b\"],\"version\":\"1.0\"}"
  Subsistema mecánico completo : Subsystem
  Subsistema térmico : Subsystem
  Sum : Sum  Inputs=++|
  TD_PARK : MATLAB Function  TreatAsAtomicUnit=on
  TI_PARK : MATLAB Function  TreatAsAtomicUnit=on
  theta_m : Outport
  T_s : Outport  Port=2
  i_abcs : Outport  Port=3
  T_m : Outport  Port=4
  omega_m : Outport  Port=5
  T_l : Outport  Port=6
  wires:
  Subsistema electromagnético/4(T_m) -> T_m/1, Subsistema mecánico completo/1(T_m)
  Subsistema electromagnético/3(i_0s) -> Subsistema térmico/3(i_0s^r), TI_PARK/3(f0s)
  Subsistema mecánico completo/2(omega_m(t)) -> Subsistema electromagnético/5(omega_m), Scope/1, omega_m/1
  Subsistema electromagnético/1(i_qs^r) -> Subsistema térmico/1(i_qs^r), TI_PARK/1(fqs)
  Subsistema electromagnético/2(i_ds^r) -> Subsistema térmico/2(i_ds^r), TI_PARK/2(fds)
  Sum/1 -> T_l/1, Subsistema mecánico completo/2(T_l)  "T_l"
  TD_PARK/1(fqs) -> Subsistema electromagnético/1(v_qs^r)
  Tº_amb/1 -> Subsistema térmico/4(Tº_amb)
  Mux/1 -> i_abcs/1
  TI_PARK/1(fas) -> Mux/1
  TI_PARK/2(fbs) -> Mux/2
  TI_PARK/3(fcs) -> Mux/3
  v_as/1 -> TD_PARK/1(fas)
  v_cs/1 -> TD_PARK/3(fcs)
  Gain/1 -> TI_PARK/4(theta_r), TD_PARK/4(theta_r)
  v_bs/1 -> TD_PARK/2(fbs)
  Gain1/1 -> Sin/1
  Sin/1 -> Gain2/1
  Gain2/1 -> Sum/1
  T_per/1 -> Sum/2
  TD_PARK/2(fds) -> Subsistema electromagnético/2(v_ds^r)
  TD_PARK/3(f0s) -> Subsistema electromagnético/3(v_0s)
  Subsistema térmico/1(r_s) -> Subsistema electromagnético/4(r_s)
  Subsistema térmico/2(T_s) -> T_s/1
  Subsistema mecánico completo/1(theta_m(t)) -> theta_m/1, Gain1/1, Gain/1
